simulink model "CommandePWM_Mesure"  (R2024b)
settings: Solver=FixedStepAuto  StartTime=0.0  StopTime=inf  RelTol=1e-3  EnableMultiTasking=on
libraries: arduinolib x2
settings Model: ExtModeTrigDuration=2  Creator=xpess  LastModifiedBy=xpess
settings OptimizationCC: EnhancedBackFolding=on  PassReuseOutputArgsAs=Individual arguments  ZeroExternalMemoryAtStartup=off  ZeroInternalMemoryAtStartup=off  MaxStackSize=64  OptimizeBlockOrder=speed  DifferentSizesBufferReuse=on  OptimizationCustomize=off  EfficientTunableParamExpr=on
settings DebuggingCC: ParameterTunabilityLossMsg=error  UnconnectedInputMsg=warning  UnconnectedOutputMsg=warning  UnconnectedLineMsg=warning
settings HardwareCC: ProdBitPerInt=16  ProdBitPerPointer=16  ProdBitPerSizeT=16  ProdBitPerPtrDiffT=16  ProdLargestAtomicFloat=None  ProdWordSize=8  ProdHWDeviceType=Atmel->AVR
settings ModelReferenceCC: EnableRefExpFcnMdlSchedulingChecks=on
settings SFSimCC: MATLABDynamicMemAlloc=off
settings RTWCC: Description=Embedded Coder  SystemTargetFile=ert.tlc  HardwareBoard=Arduino Mega 2560  TemplateMakefile=ert_default_tmf  Toolchain=Arduino AVR  BuildConfiguration=Faster Runs  GPUComputeCapability=3.5  DLArmComputeVersion=19.05
settings CodeAppCC: ForceParamTrailComments=on  IgnoreCustomStorageClasses=off  OperatorAnnotations=on  SimulinkDataObjDesc=on  SFDataObjDesc=on  InsertBlockDesc=on
settings ERTTargetCC: SupportContinuousTime=on  SupportVariableSizeSignals=on  ExtModeTransport=3  ExtModeStaticAlloc=on  ExtModeStaticAllocSize=2048  ExtModeMexFile=ext_xcp  ExtModeIntrfLevel=Level2 - Open  InlinedParameterPlacement=Hierarchical  DynamicArrayContainerType=coder::array

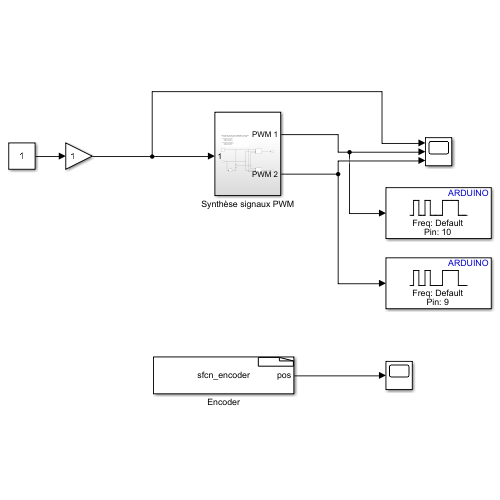
[thumbnail: Simulink's stored preview of the top-level diagram]
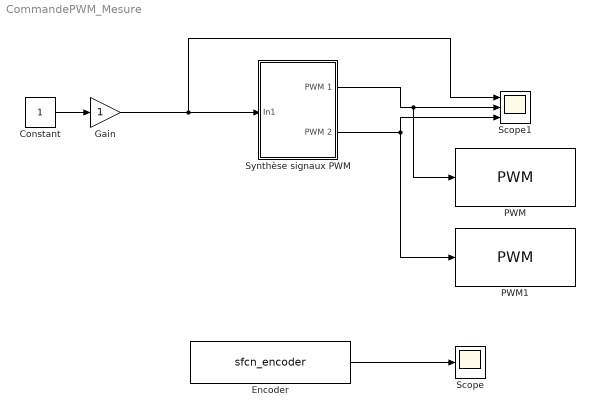
== system CommandePWM_Mesure ==
  Constant : Constant
  Encoder : S-Function  InitFcn=try, set_param(gcb,'FunctionName','sfcn_encoder'), end  FunctionName=sfcn_encoder  Parameters=uint8(0),uint8(2),uint8(13)  SFunctionModules=sfcn_encoder_wrapper  SFunctionDeploymentMode=off  EnableBusSupport=off  mask(S-Function Builder){}
      mask init:
      | val = [[.9  0.75 0.75 1 1 .9 .9 1]',[1 1 0.75 0.75 .9 .9 1 .9]'];try , sys = get_param(gcb,'SfunBuilderFcnName');if isempty(sys), sys = get_param(gcb,'FunctionName'); end,catch, sys = get_param(gcb,'FunctionName'); end
      settings: CopyFcn=set_param(gcbh,'LinkStatus','none')  PreSaveFcn=try, set_param(gcb,'FunctionName','sfcn_encoder'), end  OpenFcn=sfunctionwizard(gcbh)
      mask Display: plot(val(:,1),val(:,2)),disp(sys),port_label('output',1,'pos')
  Gain : Gain
  PWM : arduinolib/PWM  pinNumber=10  frequencyType=Default  desiredFrequency=490.2  achievableFrequency=490.2
      settings: SourceProductName=Common
  PWM1 : arduinolib/PWM  pinNumber=9  frequencyType=Default  desiredFrequency=490.2  achievableFrequency=490.2
      settings: SourceProductName=Common
  Scope : Scope
  Scope1 : Scope  NumInputPorts=3
  Synthèse signaux PWM : Subsystem
  wires:
  Gain/1 -> Scope1/1, Synthèse signaux PWM/1(In1)
  Synthèse signaux PWM/1(PWM 1) -> PWM/1, Scope1/2
  Synthèse signaux PWM/2(PWM 2) -> PWM1/1, Scope1/3
  Constant/1 -> Gain/1
  Encoder/1 -> Scope/1

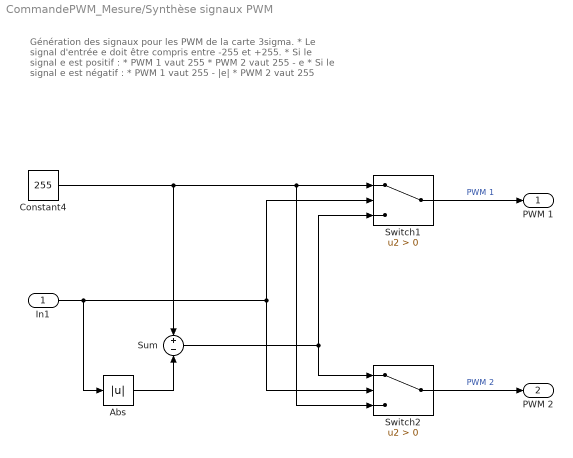
== system CommandePWM_Mesure/Synthèse signaux PWM ==
  note: Génération des signaux pour les PWM de la carte 3sigma.
      | * Le signal d'entrée e doit être compris entre -255 et +255.
      | * Si le signal e est positif :
      | * PWM 1 vaut 255
      | * PWM 2 vaut 255 - e
      | * Si le signal e est négatif :
      | * PWM 1 vaut 255 - |e|
      | * PWM 2 vaut 255
  In1 : Inport
  Abs : Abs  SaturateOnIntegerOverflow=off
  Constant4 : Constant  Value=255
  Sum : Sum  Inputs=+|-
  Switch1 : Switch  Criteria=u2 > Threshold  SaturateOnIntegerOverflow=off  InputSameDT=off
  Switch2 : Switch  Criteria=u2 > Threshold  SaturateOnIntegerOverflow=off  InputSameDT=off
  PWM 1 : Outport
  PWM 2 : Outport  Port=2
  wires:
  Constant4/1 -> Sum/1, Switch2/3, Switch1/1
  Abs/1 -> Sum/2
  Switch1/1 -> PWM 1/1  "PWM 1"
  In1/1 -> Switch1/2, Switch2/2, Abs/1
  Switch2/1 -> PWM 2/1  "PWM 2"
  Sum/1 -> Switch1/3, Switch2/1
